simulink subsystem "EnergyConvert"  (R2023b)
settings: Solver=VariableStepAuto  StartTime=0.0  StopTime=10.0  RelTol=1e-3
settings Model: Creator=mrrom  LastModifiedBy=mrrom

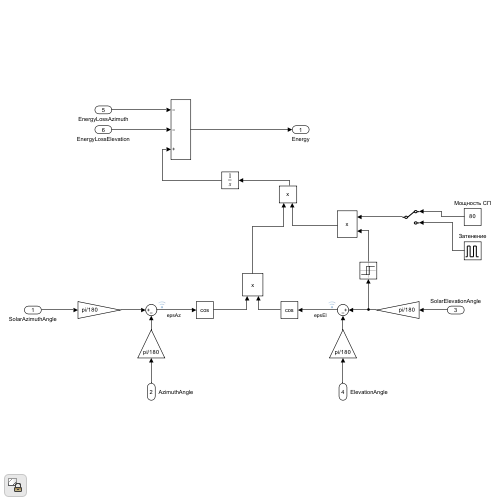
[thumbnail: Simulink's stored preview of the top-level diagram]
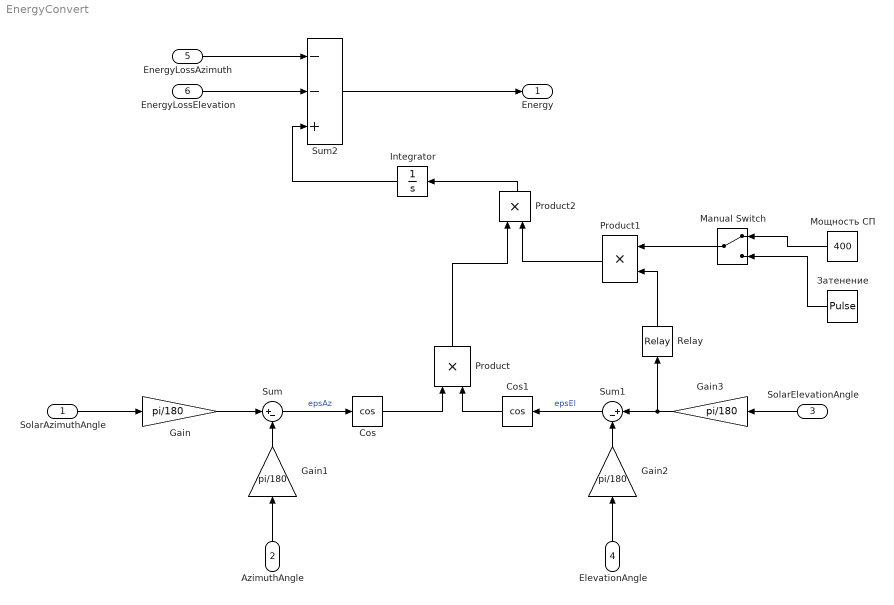
== system EnergyConvert ==
  SolarAzimuthAngle : Inport
  AzimuthAngle : Inport  Port=2
  SolarElevationAngle : Inport  Port=3
  ElevationAngle : Inport  Port=4
  EnergyLossAzimuth : Inport  Port=5
  EnergyLossElevation : Inport  Port=6
  Cos : Trigonometry  Operator=cos
  Cos1 : Trigonometry  Operator=cos
  Gain{,1..3} (4 alike) : Gain  Gain=pi/180
  Integrator : Integrator
  Manual Switch : ManualSwitch
  Product : Product
  Product1 : Product
  Product2 : Product
  Relay : Relay  OnSwitchValue=0.15  OffSwitchValue=0
  Sum : Sum  Inputs=|+-
  Sum1 : Sum  Inputs=|+-
  Sum2 : Sum  Inputs=--+
  Затенение : DiscretePulseGenerator  PulseType=Time based  Period=10  PulseWidth=5
  Мощность СП : Constant  Value=400
  Energy : Outport
  wires:
  ElevationAngle/1 -> Gain2/1
  SolarElevationAngle/1 -> Gain3/1
  Sum1/1 -> Cos1/1  "epsEl"
  SolarAzimuthAngle/1 -> Gain/1
  AzimuthAngle/1 -> Gain1/1
  Cos1/1 -> Product/2
  Cos/1 -> Product/1
  Product/1 -> Product2/1
  Sum/1 -> Cos/1  "epsAz"
  Relay/1 -> Product1/2
  Gain/1 -> Sum/1
  Gain1/1 -> Sum/2
  Gain2/1 -> Sum1/2
  Gain3/1 -> Relay/1, Sum1/1
  Product2/1 -> Integrator/1
  Product1/1 -> Product2/2
  EnergyLossAzimuth/1 -> Sum2/1
  EnergyLossElevation/1 -> Sum2/2
  Integrator/1 -> Sum2/3
  Sum2/1 -> Energy/1
  Manual Switch/1 -> Product1/1
  Мощность СП/1 -> Manual Switch/1
  Затенение/1 -> Manual Switch/2
